simulink model "control"  (R2016a)
settings: Solver=VariableStepAuto  StartTime=0.0  StopTime=7  FixedStep=0.005  RelTol=1e-3
PreLoadFcn:
  | load('param.mat')
undefined symbols (not defined in the file): a, G, Jw, M, r, T_lpf1, T_lpf2, tc
libraries: LibrarySimulinkSAS x5, simulink x4, realtime_pacer_lib x1
settings Model: Creator=M  LastModifiedBy=M

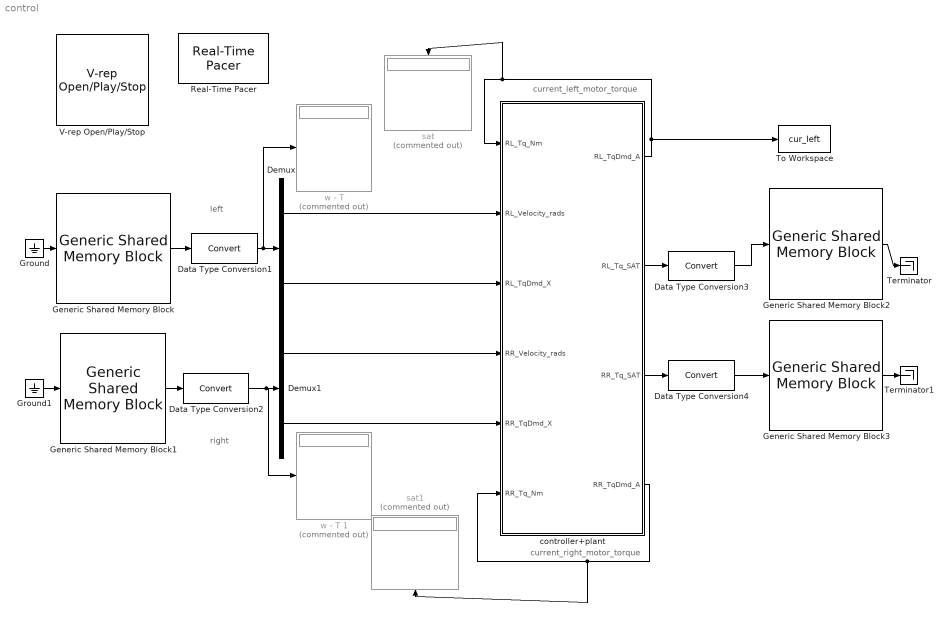
== system control ==
  note: right
  note: left
  note: current_left_motor_torque
  note: current_right_motor_torque
  Data Type Conversion{1..4} (4 alike) : DataTypeConversion
  Demux : Demux  Outputs=2
  Demux1 : Demux  Outputs=2
  Generic Shared Memory Block : LibrarySimulinkSAS/Generic Shared Memory Block  nombre='get_left'  dispositivo=2  vecE=[1]  vecS=[2]  tipoE=['f']  tipoS=['f']  ts=-1
  Generic Shared Memory Block1 : LibrarySimulinkSAS/Generic Shared Memory Block  nombre='get_right'  dispositivo=4  vecE=[1]  vecS=[2]  tipoE=['f']  tipoS=['f']  ts=-1
  Generic Shared Memory Block2 : LibrarySimulinkSAS/Generic Shared Memory Block  nombre='set_left'  dispositivo=1  vecE=[1]  vecS=[1]  tipoE=['f']  tipoS=['f']  ts=-1
  Generic Shared Memory Block3 : LibrarySimulinkSAS/Generic Shared Memory Block  nombre='set_right'  dispositivo=3  vecE=[1]  vecS=[1]  tipoE=['f']  tipoS=['f']  ts=-1
  Ground : Ground
  Ground1 : Ground
  Real-Time Pacer : realtime_pacer_lib/Real-Time Pacer  simTimePerRealTime=1
  Terminator : Terminator
  Terminator1 : Terminator
  To Workspace : ToWorkspace  VariableName=cur_left  SaveFormat=Timeseries  SampleTime=-1
  V-rep Open/Play/Stop : LibrarySimulinkSAS/V-rep Open//Play//Stop  scene='cuboidVrep.ttt'
  controller+plant : Subsystem
  sat : Display  Commented=on
  sat1 : Display  Commented=on
  w - T : Display  Commented=on
  w - T 1 : Display  Commented=on
  wires:
  controller+plant/4(RR_TqDmd_A) -> sat1/1, controller+plant/6(RR_Tq_Nm)
  Demux/1 -> controller+plant/2(RL_Velocity_rads)
  Demux/2 -> controller+plant/3(RL_TqDmd_X)
  Generic Shared Memory Block/1 -> Data Type Conversion1/1
  Data Type Conversion1/1 -> Demux/1, w - T/1
  Ground/1 -> Generic Shared Memory Block/1
  Generic Shared Memory Block1/1 -> Data Type Conversion2/1
  Data Type Conversion2/1 -> w - T 1/1, Demux1/1
  Ground1/1 -> Generic Shared Memory Block1/1
  Demux1/1 -> controller+plant/4(RR_Velocity_rads)
  Demux1/2 -> controller+plant/5(RR_TqDmd_X)
  Generic Shared Memory Block2/1 -> Terminator/1
  Generic Shared Memory Block3/1 -> Terminator1/1
  Data Type Conversion3/1 -> Generic Shared Memory Block2/1
  Data Type Conversion4/1 -> Generic Shared Memory Block3/1
  controller+plant/1(RL_TqDmd_A) -> controller+plant/1(RL_Tq_Nm), sat/1, To Workspace/1
  controller+plant/2(RL_Tq_SAT) -> Data Type Conversion3/1
  controller+plant/3(RR_Tq_SAT) -> Data Type Conversion4/1

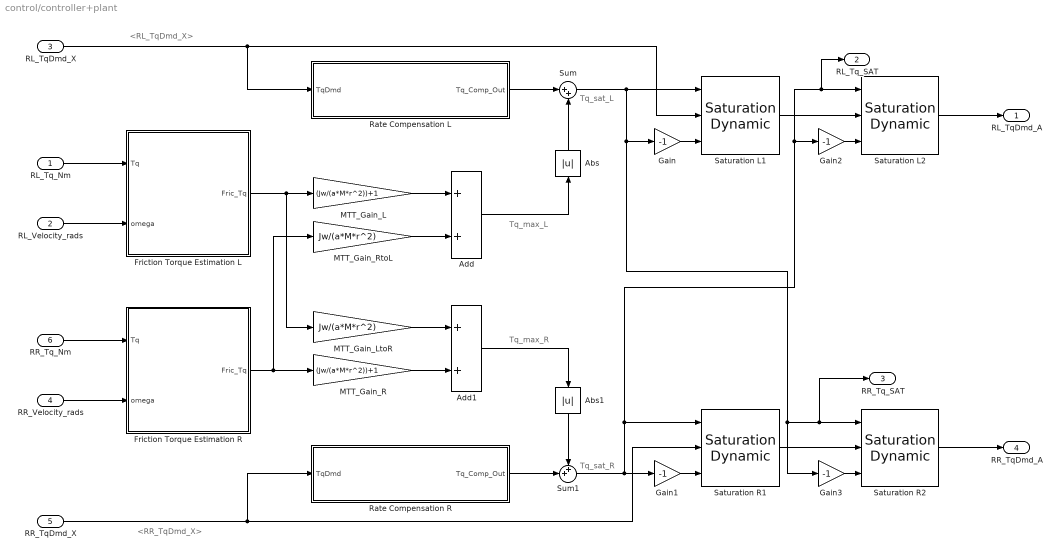
== system control/controller+plant ==
  note: Tq_sat_L
  note: Tq_sat_R
  note: Tq_max_R
  note: Tq_max_L
  note: <RR_TqDmd_X>
  note: <RL_TqDmd_X>
  RL_Tq_Nm : Inport
  RL_Velocity_rads : Inport  Port=2
  RL_TqDmd_X : Inport  Port=3
  RR_Velocity_rads : Inport  Port=4
  RR_TqDmd_X : Inport  Port=5
  RR_Tq_Nm : Inport  Port=6
  Abs : Abs  ZeroCross=off
  Abs1 : Abs  ZeroCross=off
  Add : Sum
  Add1 : Sum
  Friction Torque Estimation L : Subsystem
  Friction Torque Estimation R : Subsystem
  Gain{,1..3} (4 alike) : Gain  Gain=-1
  MTT_Gain_L : Gain  Gain=(Jw/(a*M*r^2))+1
  MTT_Gain_LtoR : Gain  Gain=Jw/(a*M*r^2)
  MTT_Gain_R : Gain  Gain=(Jw/(a*M*r^2))+1
  MTT_Gain_RtoL : Gain  Gain=Jw/(a*M*r^2)
  Rate Compensation L : Subsystem
  Rate Compensation R : Subsystem
  Saturation L1 : simulink/Discontinuities/Saturation Dynamic  OutMin=[]  OutMax=[]  OutDataTypeStr=Inherit: Same as second input  OutDataType=fixdt(1, 16)  OutScaling=2^-10  DoSatur=off
  Saturation L2 : simulink/Discontinuities/Saturation Dynamic  OutMin=[]  OutMax=[]  OutDataTypeStr=Inherit: Same as second input  OutDataType=fixdt(1, 16)  OutScaling=2^-10  DoSatur=off
  Saturation R1 : simulink/Discontinuities/Saturation Dynamic  OutMin=[]  OutMax=[]  OutDataTypeStr=Inherit: Same as second input  OutDataType=fixdt(1, 16)  OutScaling=2^-10  DoSatur=off
  Saturation R2 : simulink/Discontinuities/Saturation Dynamic  OutMin=[]  OutMax=[]  OutDataTypeStr=Inherit: Same as second input  OutDataType=fixdt(1, 16)  OutScaling=2^-10  DoSatur=off
  Sum : Sum  Inputs=|++
  Sum1 : Sum  Inputs=++|
  RL_TqDmd_A : Outport
  RL_Tq_SAT : Outport  Port=2
  RR_Tq_SAT : Outport  Port=3
  RR_TqDmd_A : Outport  Port=4
  wires:
  RL_Velocity_rads/1 -> Friction Torque Estimation L/2(omega)
  RL_Tq_Nm/1 -> Friction Torque Estimation L/1(Tq)
  RL_TqDmd_X/1 -> Saturation L1/2, Rate Compensation L/1(TqDmd)
  RR_Tq_Nm/1 -> Friction Torque Estimation R/1(Tq)
  RR_Velocity_rads/1 -> Friction Torque Estimation R/2(omega)
  RR_TqDmd_X/1 -> Saturation R1/2, Rate Compensation R/1(TqDmd)
  Friction Torque Estimation L/1(Fric_Tq) -> MTT_Gain_LtoR/1, MTT_Gain_L/1
  MTT_Gain_L/1 -> Add/1
  MTT_Gain_RtoL/1 -> Add/2
  MTT_Gain_LtoR/1 -> Add1/1
  MTT_Gain_R/1 -> Add1/2
  Friction Torque Estimation R/1(Fric_Tq) -> MTT_Gain_RtoL/1, MTT_Gain_R/1
  Add/1 -> Abs/1
  Abs/1 -> Sum/2
  Rate Compensation L/1(Tq_Comp_Out) -> Sum/1
  Add1/1 -> Abs1/1
  Rate Compensation R/1(Tq_Comp_Out) -> Sum1/2
  Abs1/1 -> Sum1/1
  Sum/1 -> Gain/1, RR_Tq_SAT/1, Saturation R2/1, Gain3/1, Saturation L1/1
  Gain/1 -> Saturation L1/3
  Gain1/1 -> Saturation R1/3
  Saturation R1/1 -> Saturation R2/2
  Saturation L1/1 -> Saturation L2/2
  Gain2/1 -> Saturation L2/3
  Sum1/1 -> Gain1/1, Saturation R1/1, Gain2/1, RL_Tq_SAT/1, Saturation L2/1
  Gain3/1 -> Saturation R2/3
  Saturation L2/1 -> RL_TqDmd_A/1
  Saturation R2/1 -> RR_TqDmd_A/1

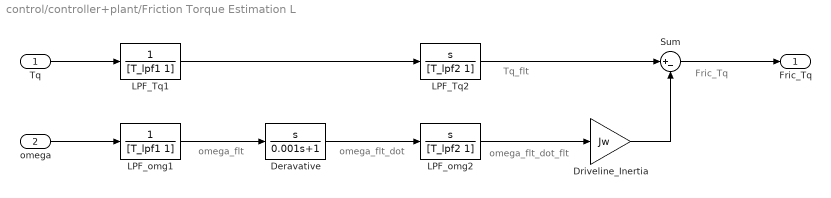
== system control/controller+plant/Friction Torque Estimation L ==
  note: omega_flt
  note: omega_flt_dot
  note: omega_flt_dot_flt
  note: Tq_flt
  note: Fric_Tq
  Tq : Inport
  omega : Inport  Port=2
  Deravative : TransferFcn  Numerator=[1 0]  Denominator=[0.001 1]
  Driveline_Inertia : Gain  Gain=Jw
  LPF_Tq1 : TransferFcn  Denominator=[T_lpf1 1]
  LPF_Tq2 : TransferFcn  Numerator=[1 0]  Denominator=[T_lpf2 1]
  LPF_omg1 : TransferFcn  Denominator=[T_lpf1 1]
  LPF_omg2 : TransferFcn  Numerator=[1 0]  Denominator=[T_lpf2 1]
  Sum : Sum  Inputs=|+-
  Fric_Tq : Outport
  wires:
  LPF_omg2/1 -> Driveline_Inertia/1
  LPF_Tq1/1 -> LPF_Tq2/1
  Deravative/1 -> LPF_omg2/1
  Driveline_Inertia/1 -> Sum/2
  LPF_Tq2/1 -> Sum/1
  Sum/1 -> Fric_Tq/1
  LPF_omg1/1 -> Deravative/1
  Tq/1 -> LPF_Tq1/1
  omega/1 -> LPF_omg1/1

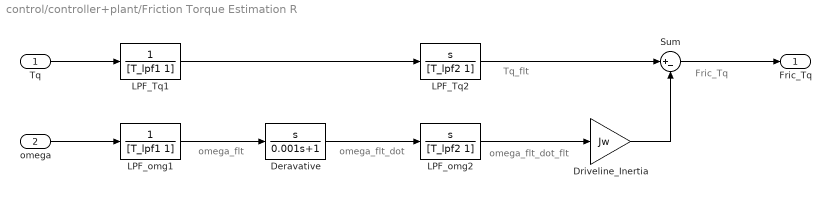
== system control/controller+plant/Friction Torque Estimation R ==
  note: omega_flt
  note: omega_flt_dot
  note: omega_flt_dot_flt
  note: Tq_flt
  note: Fric_Tq
  Tq : Inport
  omega : Inport  Port=2
  Deravative : TransferFcn  Numerator=[1 0]  Denominator=[0.001 1]
  Driveline_Inertia : Gain  Gain=Jw
  LPF_Tq1 : TransferFcn  Denominator=[T_lpf1 1]
  LPF_Tq2 : TransferFcn  Numerator=[1 0]  Denominator=[T_lpf2 1]
  LPF_omg1 : TransferFcn  Denominator=[T_lpf1 1]
  LPF_omg2 : TransferFcn  Numerator=[1 0]  Denominator=[T_lpf2 1]
  Sum : Sum  Inputs=|+-
  Fric_Tq : Outport
  wires:
  LPF_omg2/1 -> Driveline_Inertia/1
  LPF_Tq1/1 -> LPF_Tq2/1
  Deravative/1 -> LPF_omg2/1
  Driveline_Inertia/1 -> Sum/2
  LPF_Tq2/1 -> Sum/1
  Sum/1 -> Fric_Tq/1
  LPF_omg1/1 -> Deravative/1
  Tq/1 -> LPF_Tq1/1
  omega/1 -> LPF_omg1/1

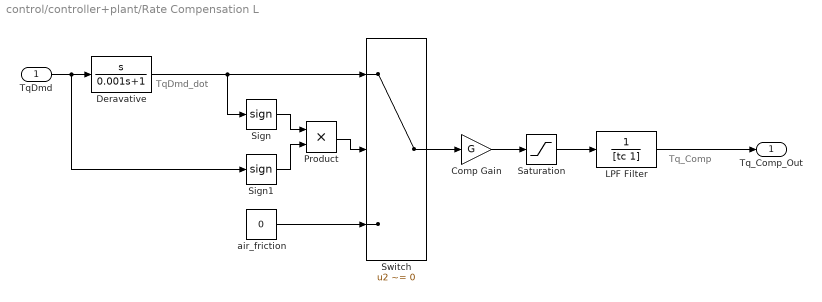
== system control/controller+plant/Rate Compensation L ==
  note: Tq_Comp
  note: TqDmd_dot
  TqDmd : Inport
  Comp Gain : Gain  Gain=G
  Deravative : TransferFcn  Numerator=[1 0]  Denominator=[0.001 1]
  LPF Filter : TransferFcn  Denominator=[tc 1]
  Product : Product
  Saturation : Saturate  UpperLimit=500  LowerLimit=0  ZeroCross=off
  Sign : Signum
  Sign1 : Signum
  Switch : Switch  Criteria=u2 ~= 0
  "air_friction " : Constant  Value=0
  Tq_Comp_Out : Outport
  wires:
  TqDmd/1 -> Sign1/1, Deravative/1
  "air_friction "/1 -> Switch/3
  Sign1/1 -> Product/2
  Sign/1 -> Product/1
  Product/1 -> Switch/2
  Switch/1 -> Comp Gain/1
  Saturation/1 -> LPF Filter/1
  Comp Gain/1 -> Saturation/1
  LPF Filter/1 -> Tq_Comp_Out/1
  Deravative/1 -> Switch/1, Sign/1

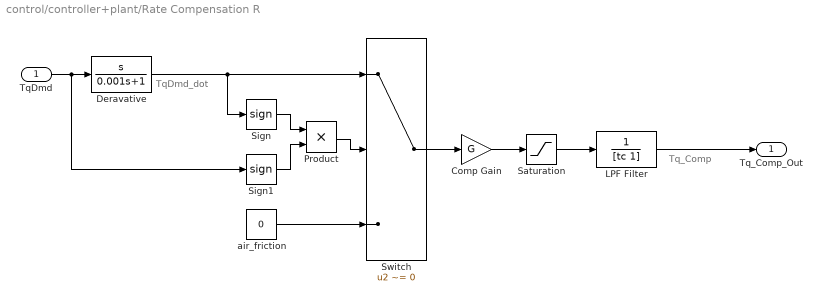
== system control/controller+plant/Rate Compensation R ==
  note: TqDmd_dot
  note: Tq_Comp
  TqDmd : Inport
  Comp Gain : Gain  Gain=G
  Deravative : TransferFcn  Numerator=[1 0]  Denominator=[0.001 1]
  LPF Filter : TransferFcn  Denominator=[tc 1]
  Product : Product
  Saturation : Saturate  UpperLimit=500  LowerLimit=0  ZeroCross=off
  Sign : Signum
  Sign1 : Signum
  Switch : Switch  Criteria=u2 ~= 0
  air_friction : Constant  Value=0
  Tq_Comp_Out : Outport
  wires:
  Deravative/1 -> Sign/1, Switch/1
  LPF Filter/1 -> Tq_Comp_Out/1
  Comp Gain/1 -> Saturation/1
  Saturation/1 -> LPF Filter/1
  Switch/1 -> Comp Gain/1
  Product/1 -> Switch/2
  Sign/1 -> Product/1
  Sign1/1 -> Product/2
  air_friction/1 -> Switch/3
  TqDmd/1 -> Deravative/1, Sign1/1
